simulink subsystem "suspension_ss"  (R2022a)
settings: Solver=VariableStepAuto  StartTime=0.0  StopTime=10.0  RelTol=1e-3
model mask{obj=slPart}
  mask prompts: obj "slPart Object:"
settings Model: Creator=grouleau  LastModifiedBy=grouleau

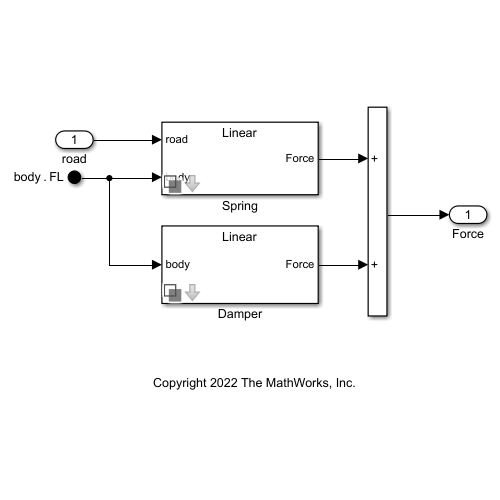
[thumbnail: Simulink's stored preview of the top-level diagram]
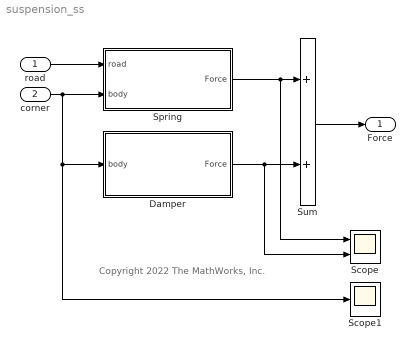
== system suspension_ss ==
  note: Copyright 2022 The MathWorks, Inc.
  road : Inport
  corner : Inport  Port=2
  Damper : Subsystem  Variant=on  VariantControlMode=label  LabelModeActiveChoice=damper.linear  mask(slPart){obj=obj.Damper}
      mask prompts: obj "slPart Object:"
      mask help: Container block for all slPart blocks
      mask init:
      | obj.maskInit(gcb);
  Scope : Scope  NumInputPorts=2
  Scope1 : Scope
  Spring : Subsystem  Variant=on  VariantControlMode=label  LabelModeActiveChoice=spring.linear  mask(slPart){obj=obj.Spring}
      mask prompts: obj "slPart Object:"
      mask help: Container block for all slPart blocks
      mask init:
      | obj.maskInit(gcb);
  Sum : Sum
  Force : Outport
  wires:
  corner/1 -> Damper/1(body), Scope1/1, Spring/2(body)
  Spring/1(Force) -> Sum/1, Scope/1
  road/1 -> Spring/1(road)
  Damper/1(Force) -> Sum/2, Scope/2
  Sum/1 -> Force/1

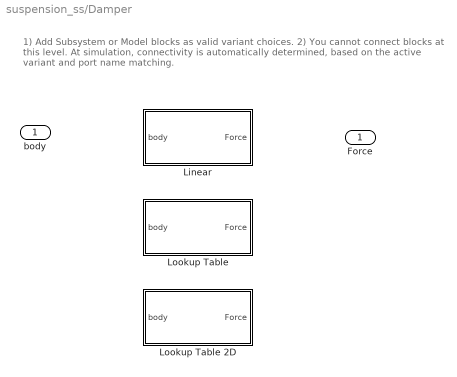
== system suspension_ss/Damper ==
  note: 1) Add Subsystem or Model blocks as valid variant choices.
      | 2) You cannot connect blocks at this level. At simulation, connectivity is automatically
      | determined, based on the active variant and port name matching.
  body : Inport
  Linear : Subsystem  VariantControl=damper.linear
  Lookup Table : Subsystem  VariantControl=damper.lookup
  Lookup Table 2D : Subsystem  VariantControl=damper.lookup2D
  Force : Outport

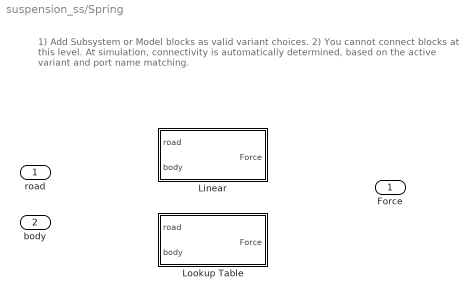
== system suspension_ss/Spring ==
  note: 1) Add Subsystem or Model blocks as valid variant choices.
      | 2) You cannot connect blocks at this level. At simulation, connectivity is automatically
      | determined, based on the active variant and port name matching.
  road : Inport
  body : Inport  Port=2
  Linear : Subsystem  VariantControl=spring.linear
  Lookup Table : Subsystem  VariantControl=spring.lookup
  Force : Outport

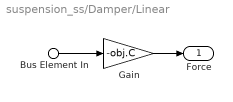
== system suspension_ss/Damper/Linear ==
  Bus Element In : Inport  PortName=body  Element=zDot
  Gain : Gain  Gain=-obj.C
  Force : Outport
  wires:
  Bus Element In/1 -> Gain/1
  Gain/1 -> Force/1

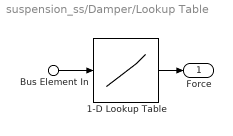
== system suspension_ss/Damper/Lookup Table ==
  Bus Element In : Inport  PortName=body  Element=zDot
  1-D Lookup Table : Lookup_n-D  NumberOfTableDimensions=1  BreakpointsForDimension1=obj.dx  Table=obj.C  InternalRulePriority=Speed  RndMeth=Simplest
  Force : Outport
  wires:
  1-D Lookup Table/1 -> Force/1
  Bus Element In/1 -> 1-D Lookup Table/1

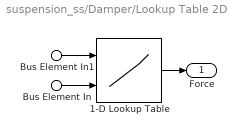
== system suspension_ss/Damper/Lookup Table 2D ==
  Bus Element In : Inport  PortName=body  Element=zDot
  Bus Element In1 : Inport  PortName=body  Element=z
  1-D Lookup Table : Lookup_n-D  BreakpointsForDimension1=obj.x  BreakpointsForDimension2=obj.dx  Table=obj.C  InternalRulePriority=Speed  RndMeth=Simplest
      settings: InputPortMap=u0,u1
  Force : Outport
  wires:
  Bus Element In1/1 -> 1-D Lookup Table/1
  Bus Element In/1 -> 1-D Lookup Table/2
  1-D Lookup Table/1 -> Force/1

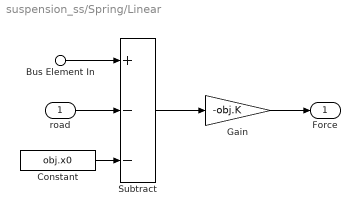
== system suspension_ss/Spring/Linear ==
  road : Inport
  Bus Element In : Inport  Port=2  PortName=body  Element=z
  Constant : Constant  Value=obj.x0
  Gain : Gain  Gain=-obj.K
  Subtract : Sum  Inputs=+--
  Force : Outport
  wires:
  Bus Element In/1 -> Subtract/1
  road/1 -> Subtract/2
  Constant/1 -> Subtract/3
  Subtract/1 -> Gain/1
  Gain/1 -> Force/1

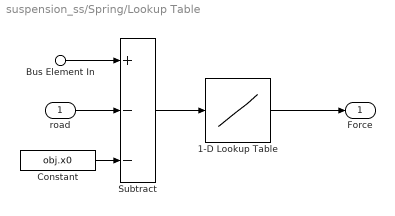
== system suspension_ss/Spring/Lookup Table ==
  road : Inport
  Bus Element In : Inport  Port=2  PortName=body  Element=z
  1-D Lookup Table : Lookup_n-D  NumberOfTableDimensions=1  BreakpointsForDimension1=obj.x  Table=obj.K  InternalRulePriority=Speed  RndMeth=Simplest
  Constant : Constant  Value=obj.x0
  Subtract : Sum  Inputs=+--
  Force : Outport
  wires:
  1-D Lookup Table/1 -> Force/1
  Subtract/1 -> 1-D Lookup Table/1
  Constant/1 -> Subtract/3
  road/1 -> Subtract/2
  Bus Element In/1 -> Subtract/1
